simulink model "METI_CVT_Thermal_ver01_2015a"  (R2015a)
settings: Solver=ode8  SolverMode=SingleTasking  StartTime=0  StopTime=1204  FixedStep=sampling_time  RelTol=1e-3
PreLoadFcn:
  | init_setting;
values from neighbouring files (symbols this model uses):
  degC2K = 273.15    [METI_TRAMI_Thermal_ver01_Jmaab_PreLoad.m]    (also in init_setting_METI.m)
  K2degC = -273.15    [METI_TRAMI_Thermal_ver01_Jmaab_PreLoad.m]    (also in init_setting_METI.m)
  sampling_time = 0.0025    [METI_TRAMI_Thermal_ver01_Jmaab_PreLoad.m]
undefined symbols (not defined in the file or in its folder): ALT_CNT_ALT_OFF_RPM_HYS_rpm, ALT_CNT_ALT_ON_RPM_HYS_rpm, ALT_CNT_Alter_V_BASE_V, ALT_CNT_Alter_V_Kaisei_V, ALT_CNT_flag_disable_kaisei, ALT_CNT_V_Battely_Kudo_V, ALT_PNT_ALT_GDCurrent_A, ALT_PNT_ALT_GDVolt_V, ALT_PNT_Alter_limit_Current_V_table, ALT_PNT_Alter_limit_Current_V_table_x_rpm, ALT_PNT_Alter_trq_Nm_map, ALT_PNT_Alter_trq_Nm_map_x_rpm, ALT_PNT_Alter_trq_Nm_map_y_Current_A, ALT_PNT_Alter_trq_Nm_map_z_Volt_tgt_V, ALT_PNT_eta_pulley_alt, ALT_PNT_Gain_Alt_v_del, ALT_PNT_ratio_pulley_alt, ALT_PNT_Tau_Alternator_V_tgt_s, ALT_PNT_trq_alter_output_LL_Nm, BK_PNT_Pow_UL, BK_PNT_Tau_brake, Brk_LL, Brk_PGain, Brk_UL, BT_PNT_Lo_Capa_lo_batt_F, BT_PNT_Lo_ocv_SOC_lo_batt_OCV_V_table, BT_PNT_Lo_ocv_SOC_lo_batt_OCV_V_table_x_SOC, BT_PNT_Lo_R_lo_batt_ohm, BT_PNT_Lo_SOC_MAX_lo_batt, BT_PNT_Lo_SOC_MIN_lo_batt, BT_PNT_Lo_SOC_START_lo_batt, DF_PNT_DF_gear, DF_PNT_DFBlock2DFAir_Heat_Resi_KpW, DF_PNT_DFBlock_Heat_Capa_JpK, DF_PNT_DFBlock_Temp_ini_degC, DF_PNT_DFOil2DFBlock_Heat_Resi_KpW, DF_PNT_DFOil_Heat_Capa_JpK, DF_PNT_DFOil_Temp_ini_degC, DF_PNT_Driveshaft_damper, DF_PNT_Driveshaft_delta_radps_LL, DF_PNT_Driveshaft_delta_radps_UL, DF_PNT_Driveshaft_spring, DF_PNT_eta_DF, DF_PNT_Outtemp_degC, DF_PNT_TMBlock2DFBlock_Heat_Resi_KpW, Driver_Brake_Const1, Driver_Brake_Const3, Driver_Brake_Switch_Const2, Driver_Brk_sh, drivmode_ACC, drivmode_CONST, drivmode_GensokuKaisei, drivmode_GensokuRikko, drivmode_STOP, EL_PNT_R_bodyelec_lo_ohm, ENG_CNT_acc_idlestop, ENG_CNT_Accel_LL, ENG_CNT_Accel_UL, ENG_CNT_brak_idlestop, ENG_CNT_flag_idle_stop_exe ... (+133)
undefined symbols (not defined in the file): ACC_D_Gain, ACC_I_Gain, ACC_P_Gain
libraries: METI_Lib_vehicle_model x32, simulink x7, AZAPA_Lib_vehicle_model x1
(part 3 of 3)

== system METI_CVT_Thermal_ver01_2015a/Vehicle/TM_PNT/TC_PNT ==
  note: ロックアップクラッチ
  note: トルクコンバータ
  flag_Lockup : Inport
  omg_Slip_rpm : Inport  Port=2
  w_TM_PNT_in_radps : Inport  Port=3
  w_TM_PNT_in_radps2 : Inport  Port=4
  Gain : Gain  Gain=-1
  LU_Clutch : Subsystem
  P_cal : METI_Lib_vehicle_model/P_cal  Type_energy=回転運動  Type_output_energy=出力  Power_name=Po_  t_Workspace_Name=TM_PNT_TC_MECK_UP  P_VariableName=Po_TM_PNT_TC_MECK_UP  Across_VariableName=w_TM_PNT_TC_MECK_UP  Throgh_VariableName=tq_TM_PNT_TC_MECK_UP
  P_cal1 : METI_Lib_vehicle_model/P_cal  Type_energy=回転運動  Type_output_energy=出力  Power_name=Po_  t_Workspace_Name=TM_PNT_TC_MECK_DN  P_VariableName=Po_TM_PNT_TC_MECK_DN  Across_VariableName=w_TM_PNT_TC_MECK_DN  Throgh_VariableName=tq_TM_PNT_TC_MECK_DN
  P_cal2 : METI_Lib_vehicle_model/P_cal  Type_energy=回転運動  Type_output_energy=出力  Power_name=Po_  t_Workspace_Name=TM_PNT_LU_MECK_UP  P_VariableName=Po_TM_PNT_LU_MECK_UP  Across_VariableName=w_TM_PNT_LU_MECK_UP  Throgh_VariableName=tq_TM_PNT_LU_MECK_UP
  P_cal3 : METI_Lib_vehicle_model/P_cal  Type_energy=回転運動  Type_output_energy=出力  Power_name=Po_  t_Workspace_Name=TM_PNT_LU_MECK_DN  P_VariableName=Po_TM_PNT_LU_MECK_DN  Across_VariableName=w_TM_PNT_LU_MECK_DN  Throgh_VariableName=tq_TM_PNT_LU_MECK_DN
  Sum : Sum  Inputs=|++
  Sum1 : Sum  Inputs=|++
  T_C : Subsystem
  Terminator{,1..4} (5 alike) : Terminator
  trq_TM_PNT_in_Nm2 : Outport
  trq_TM_PNT_in_Nm1 : Outport  Port=2
  wires:
  T_C/2(trq_TC_Nm2) -> Sum/2, P_cal/2
  w_TM_PNT_in_radps/1 -> T_C/1(w_TM_PNT_in_radps1), P_cal/1, LU_Clutch/2(w_TM_PNT_in_radps1), P_cal2/1
  Sum/1 -> Gain/1
  T_C/1(trq_TC_Nm1) -> P_cal1/2, Sum1/2
  Sum1/1 -> trq_TM_PNT_in_Nm2/1
  w_TM_PNT_in_radps2/1 -> LU_Clutch/3(w_TM_PNT_in_radps2), P_cal1/1, P_cal3/1, T_C/2(w_TM_PNT_in_radps2)
  P_cal/1 -> Terminator/1
  P_cal1/1 -> Terminator1/1
  omg_Slip_rpm/1 -> Terminator3/1
  LU_Clutch/1(trq_LUC_Nm1) -> Sum/1, P_cal2/2
  LU_Clutch/2(trq_LUC_Nm2) -> Sum1/1, P_cal3/2
  flag_Lockup/1 -> LU_Clutch/1(LockUP_Signal)
  P_cal2/1 -> Terminator2/1
  P_cal3/1 -> Terminator4/1
  Gain/1 -> trq_TM_PNT_in_Nm1/1

== system METI_CVT_Thermal_ver01_2015a/Vehicle/TM_PNT/VR_PNT ==
  note: ギア比変換
  ratio_CVT : Inport
  trq_TM_PNT_in_Nm2 : Inport  Port=2
  w_TM_PNT_out_radps0 : Inport  Port=3
  T_TMTH_PNT_CVTF_dC : Inport  Port=4
  1-D Lookup Table : Lookup_n-D  NumberOfTableDimensions=1  BreakpointsForDimension1=TM_PNT_eta_CVT_x_CVTF_degC  Table=TM_PNT_eta_CVT  InternalRulePriority=Speed  RndMeth=Simplest  InputSameDT=on
  Goto1 : Goto  Commented=on  GotoTag=trq_Variator_Nm
  P_cal : METI_Lib_vehicle_model/P_cal  Type_energy=回転運動  Type_output_energy=損失  Power_name=Pl_  t_Workspace_Name=TM_PNT_Variator_MECK_LOSS  P_VariableName=Pl_TM_PNT_Variator_MECK_LOSS  Across_VariableName=w_TM_PNT_Variator_MECK_LOSS  Throgh_VariableName=tq_TM_PNT_Variator_MECK_LOSS
  Product : Product  RndMeth=Zero
  Product1 : Product  RndMeth=Zero
  Transfer Fcn : TransferFcn  Denominator=[TM_PNT_Tau_CVT_ratio_s 1]
  eta_cal_CVT : METI_Lib_vehicle_model/eta_cal_InHi
  trq_TM_PNT_out_Nm0 : Outport
  w_TM_PNT_in_radps2 : Outport  Port=2
  tag scope: tScope_CVTLoss=global
  wires:
  trq_TM_PNT_in_Nm2/1 -> eta_cal_CVT/2
  Product/1 -> w_TM_PNT_in_radps2/1, P_cal/1
  w_TM_PNT_out_radps0/1 -> Product/2
  ratio_CVT/1 -> Transfer Fcn/1
  Product1/1 -> Goto1/1, trq_TM_PNT_out_Nm0/1
  eta_cal_CVT/2 -> Product1/2
  P_cal/1 -> [tScope_CVTLoss]
  Transfer Fcn/1 -> Product1/1, Product/1
  1-D Lookup Table/1 -> eta_cal_CVT/1
  eta_cal_CVT/1 -> P_cal/2
  T_TMTH_PNT_CVTF_dC/1 -> 1-D Lookup Table/1

== system METI_CVT_Thermal_ver01_2015a/Driver/Caliculate_Opeining_Accel/FB/Filter ==
  In1 : Inport
  Gain3 : Gain  Gain=10
  Gain4 : Gain  Gain=0.1
  Rounding Function : Rounding  Operator=round
  Out1 : Outport
  wires:
  Rounding Function/1 -> Gain4/1
  In1/1 -> Gain3/1
  Gain3/1 -> Rounding Function/1
  Gain4/1 -> Out1/1

== system METI_CVT_Thermal_ver01_2015a/Driver/Caliculate_Opeining_Accel/FF/Air_Resistance ==
  V_tgt : Inport
  V_wind : Constant  Value=VL_PNT_V_wind
  cal_Air_resi1 : METI_Lib_vehicle_model/vehicle_model/cal_Air_resi  Vel_max=200
  F_air_resi : Outport
  wires:
  V_tgt/1 -> cal_Air_resi1/1
  V_wind/1 -> cal_Air_resi1/2
  cal_Air_resi1/1 -> F_air_resi/1

== system METI_CVT_Thermal_ver01_2015a/Driver/Caliculate_Opeining_Accel/FF/Cal_M_ENG_jiku2 ==
  note: 軸トルクマップ
  FF_trq_accel_Nm : Inport
  pre_n_eng_rpm : Inport  Port=2
  2-D Lookup Table : Lookup_n-D  BreakpointsForDimension1=ENG_trq_rev  BreakpointsForDimension2=ENG_rpm  Table=ENG_throttle_rev  ExtrapMethod=Clip  UseLastTableValue=on  RndMeth=Simplest  InputSameDT=on
  2-D Lookup Table1 : Lookup_n-D  BreakpointsForDimension1=ENG_PNT_trq_Nm_map_y_throttle  BreakpointsForDimension2=ENG_PNT_trq_Nm_map_x_rpm  Table=ENG_PNT_trq_Nm_map  ExtrapMethod=Clip  UseLastTableValue=on  RndMeth=Simplest  InputSameDT=on
  Constant : Constant  Value=0
  Subsystem : Subsystem
  Sum : Sum  Inputs=|++
  FF_open_accel_per : Outport
  wires:
  FF_trq_accel_Nm/1 -> Sum/1
  2-D Lookup Table/1 -> Subsystem/1(In1)
  pre_n_eng_rpm/1 -> 2-D Lookup Table/2, 2-D Lookup Table1/2
  Constant/1 -> 2-D Lookup Table1/1
  Sum/1 -> 2-D Lookup Table/1
  2-D Lookup Table1/1 -> Sum/2
  Subsystem/1(Out1) -> FF_open_accel_per/1

== system METI_CVT_Thermal_ver01_2015a/Driver/Caliculate_Opeining_Accel/FF/Inertial_Resistance ==
  V_tgt : Inport
  Constant : Constant  Value=M
  Derivative : Derivative
  Divide : Product  OutDataTypeStr=Inherit: Same as first input
  F_Inertia : Outport
  wires:
  Constant/1 -> Divide/2
  Derivative/1 -> Divide/1
  Divide/1 -> F_Inertia/1
  V_tgt/1 -> Derivative/1

== system METI_CVT_Thermal_ver01_2015a/Driver/Caliculate_Opeining_Accel/FF/Rolling_Resistance ==
  note: 20151211修正
      |
      | 空気抵抗と表現を統一する、ため
      | -1のGainを削除
  V_tgt : Inport
  cal_roll_resi1 : METI_Lib_vehicle_model/vehicle_model/cal_roll_resi  Myu_tire=myu  Vehicle_Mass=M  Gravi_acc=g
  F_rollresi : Outport
  wires:
  V_tgt/1 -> cal_roll_resi1/1
  cal_roll_resi1/1 -> F_rollresi/1

== system METI_CVT_Thermal_ver01_2015a/Vehicle/ALT_PNT/Subsystem/I_alt_cal ==
  target_volt_ALT_V : Inport
  volt_BT_PNT_Lo_V : Inport  Port=2
  rpm_alt : Inport  Port=3
  Add : Sum
  Cal_I_alt_P_control : Subsystem
  Cal_I_alt_base : Subsystem
  Constant : Constant  Value=12
  Constant4 : Constant  Value=0
  Limit_Current_Max : Lookup_n-D  NumberOfTableDimensions=1  BreakpointsForDimension1=ALT_PNT_Alter_limit_Current_V_table_x_rpm  Table=ALT_PNT_Alter_limit_Current_V_table  ExtrapMethod=Clip  UseLastTableValue=on  RndMeth=Simplest  InputSameDT=on
  MinMax2 : MinMax  Function=max  Inputs=2
  Sum1 : Sum  Inputs=|+-
  Sum2 : Sum  Inputs=-+|
  電圧比較 : MinMax  Inputs=2
  I_alt : Outport
  wires:
  target_volt_ALT_V/1 -> Sum1/1, Sum2/2
  volt_BT_PNT_Lo_V/1 -> Sum2/1
  rpm_alt/1 -> Limit_Current_Max/1
  Constant4/1 -> MinMax2/2
  Limit_Current_Max/1 -> MinMax2/1  "I_limit_ALT"
  電圧比較/1 -> I_alt/1
  Add/1 -> 電圧比較/2
  Sum2/1 -> Cal_I_alt_P_control/1(V_delt_tgt)
  MinMax2/1 -> 電圧比較/1
  Constant/1 -> Sum1/2
  Sum1/1 -> Cal_I_alt_base/1(V_delt_tgt)
  Cal_I_alt_P_control/1(I_alt_base) -> Add/1
  Cal_I_alt_base/1(I_alt_base) -> Add/2

== system METI_CVT_Thermal_ver01_2015a/Vehicle/ALT_PNT/Subsystem/Torque_Guard ==
  current_ALT_PNT_A : Inport
  V_ALT_PNT : Inport  Port=2
  n_ROT_slavepulley12_rpm : Inport  Port=3
  ALT_GDCurrent : Inport  Port=4
  ALT_GDVolt : Inport  Port=5
  Caliculate_Axes_Torque1 : Lookup_n-D  NumberOfTableDimensions=3  BreakpointsForDimension1=ALT_PNT_Alter_trq_Nm_map_x_rpm  BreakpointsForDimension2=ALT_PNT_Alter_trq_Nm_map_y_Current_A  BreakpointsForDimension3=ALT_PNT_Alter_trq_Nm_map_z_Volt_tgt_V  Table=ALT_PNT_Alter_trq_Nm_map  RndMeth=Simplest  InputSameDT=on
  Caliculate_Axes_Torque2 : Lookup_n-D  NumberOfTableDimensions=3  BreakpointsForDimension1=ALT_PNT_Alter_trq_Nm_map_x_rpm  BreakpointsForDimension2=ALT_PNT_Alter_trq_Nm_map_y_Current_A  BreakpointsForDimension3=ALT_PNT_Alter_trq_Nm_map_z_Volt_tgt_V  Table=ALT_PNT_Alter_trq_Nm_map  RndMeth=Simplest  InputSameDT=on
  Constant3 : Constant  Value=ALT_PNT_trq_alter_output_LL_Nm
  MinMax : MinMax  Inputs=2
  MinMax1 : MinMax  Function=max  Inputs=2
  trq_trqsource : Outport
  wires:
  ALT_GDCurrent/1 -> Caliculate_Axes_Torque2/2
  Caliculate_Axes_Torque2/1 -> MinMax/2
  MinMax/1 -> MinMax1/1
  Caliculate_Axes_Torque1/1 -> MinMax/1
  Constant3/1 -> MinMax1/2
  ALT_GDVolt/1 -> Caliculate_Axes_Torque2/3
  MinMax1/1 -> trq_trqsource/1
  V_ALT_PNT/1 -> Caliculate_Axes_Torque1/3
  current_ALT_PNT_A/1 -> Caliculate_Axes_Torque1/2
  n_ROT_slavepulley12_rpm/1 -> Caliculate_Axes_Torque2/1, Caliculate_Axes_Torque1/1

== system METI_CVT_Thermal_ver01_2015a/Vehicle/BT_LO_PNT/Cal_SOC/Subsystem4 ==
  In1 : Inport
  In2 : Inport  Port=2
  To Workspace : ToWorkspace  VariableName=SOC_LoBat  SampleTime=-1
      settings: Decimation=num_tws_mabiki
  To Workspace1 : ToWorkspace  VariableName=Asec_LoBat  SampleTime=-1
      settings: Decimation=num_tws_mabiki
  wires:
  In1/1 -> To Workspace/1
  In2/1 -> To Workspace1/1

== system METI_CVT_Thermal_ver01_2015a/Vehicle/ENG_CNT/Caliculate_Idle_Speed/Subsystem ==
  del_omg_engine : Inport
  flag_idle_fb : Inport  Port=2
  Gain : Gain  Gain=ENG_CNT_gain_p_per_isc
  Logical Operator1 : Logic  Operator=NOT  AllPortsSameDT=off  OutDataTypeStr=boolean
  Memory : Memory  X0=4
  Saturation : Saturate  UpperLimit=ENG_CNT_per_isc_max  LowerLimit=ENG_CNT_per_isc_min
  Switch : Switch  Criteria=u2 > Threshold  Threshold=0.5
  per_isc_[%] : Outport
  wires:
  Switch/1 -> Saturation/1
  flag_idle_fb/1 -> Logical Operator1/1
  Gain/1 -> Switch/3
  Memory/1 -> Switch/1
  Saturation/1 -> per_isc_[%]/1, Memory/1
  del_omg_engine/1 -> Gain/1
  Logical Operator1/1 -> Switch/2

== system METI_CVT_Thermal_ver01_2015a/Vehicle/ENG_CNT/Caliculate_Idle_Speed/Subsystem1 ==
  note: アイドル回転数時のFB
  omg_tgt_idle : Inport
  n_eng_rpm : Inport  Port=2
  per_throttle_base : Inport  Port=3
  flag_Lockup : Inport  Port=4
  flag_IdleStop : Inport  Port=5
  Logical Operator : Logic  Operator=OR  AllPortsSameDT=off  OutDataTypeStr=boolean
  Logical Operator1 : Logic  Operator=NOT  AllPortsSameDT=off  OutDataTypeStr=boolean
  Logical Operator2 : Logic  Inputs=3  AllPortsSameDT=off  OutDataTypeStr=boolean
  Logical Operator3 : Logic  Operator=NOT  AllPortsSameDT=off  OutDataTypeStr=boolean
  Logical Operator4 : Logic  Operator=NOT  AllPortsSameDT=off  OutDataTypeStr=boolean
  Logical Operator5 : Logic  AllPortsSameDT=off  OutDataTypeStr=boolean
  Relational Operator : RelationalOperator  Operator=<  OutDataTypeStr=boolean
  Relational Operator2 : RelationalOperator  Operator=>  OutDataTypeStr=boolean
  per_throttle_isc_fb : Constant  Value=ENG_CNT_per_throttle_isc_fb
  flag_idle_fb : Outport
  wires:
  per_throttle_base/1 -> Relational Operator/1
  per_throttle_isc_fb/1 -> Relational Operator/2
  Relational Operator2/1 -> Logical Operator2/1
  Relational Operator/1 -> Logical Operator1/1, Logical Operator5/1
  Logical Operator1/1 -> Logical Operator2/2
  Logical Operator5/1 -> Logical Operator/2
  flag_Lockup/1 -> Logical Operator3/1
  Logical Operator3/1 -> Logical Operator2/3
  Logical Operator2/1 -> Logical Operator/1
  omg_tgt_idle/1 -> Relational Operator2/1
  n_eng_rpm/1 -> Relational Operator2/2
  flag_IdleStop/1 -> Logical Operator4/1
  Logical Operator4/1 -> Logical Operator5/2
  Logical Operator/1 -> flag_idle_fb/1

== system METI_CVT_Thermal_ver01_2015a/Vehicle/ENG_PNT/Cal_FuelComsunption/Not_cal1 ==
  In1 : Inport
  Constant : Constant  Value=0
  Constant1 : Constant
  Switch : Switch  Criteria=u2 > Threshold  Threshold=0.5
  Out1 : Outport
  wires:
  Constant1/1 -> Switch/3
  Constant/1 -> Switch/1
  Switch/1 -> Out1/1
  In1/1 -> Switch/2

== system METI_CVT_Thermal_ver01_2015a/Vehicle/ENG_PNT/Cal_FuelComsunption/Not_cal2 ==
  In1 : Inport
  Constant : Constant  Value=0
  Constant1 : Constant
  Switch : Switch  Criteria=u2 > Threshold  Threshold=0.5
  Out1 : Outport
  wires:
  In1/1 -> Switch/2
  Switch/1 -> Out1/1
  Constant/1 -> Switch/1
  Constant1/1 -> Switch/3

== system METI_CVT_Thermal_ver01_2015a/Vehicle/ENG_PNT/Cal_trq_ENG_jiku/Not_cal ==
  In1 : Inport
  Constant : Constant  Value=0
  Constant1 : Constant
  Switch : Switch  Criteria=u2 > Threshold  Threshold=0.5
  Out1 : Outport
  wires:
  In1/1 -> Switch/2
  Switch/1 -> Out1/1
  Constant/1 -> Switch/1
  Constant1/1 -> Switch/3

== system METI_CVT_Thermal_ver01_2015a/Vehicle/ENG_PNT/Cal_trq_ENG_jiku/Not_cal1 ==
  In1 : Inport
  Constant : Constant  Value=0
  Constant1 : Constant
  Switch : Switch  Criteria=u2 > Threshold  Threshold=0.5
  Out1 : Outport
  wires:
  Constant1/1 -> Switch/3
  Constant/1 -> Switch/1
  Switch/1 -> Out1/1
  In1/1 -> Switch/2

== system METI_CVT_Thermal_ver01_2015a/Vehicle/PTTH_PNT/DFTH_PNT/DFBlock_Heat_Capacity ==
  PHI_DFBlock3_W : Inport
  PHI_DFBlock2_W : Inport  Port=2
  PHI_DFBlock1_W : Inport  Port=3
  Add : Sum  Inputs=+++
  Add1 : Sum
  Constant : Constant  Value=DF_PNT_DFBlock_Heat_Capa_JpK
  Constant1 : Constant  Value=DF_PNT_DFBlock_Temp_ini_degC
  Divide : Product  Inputs=/*
  Integrator : Integrator
  degC->K : Subsystem
  T_DFBlock2_K : Outport
  T_DFBlock3_K : Outport  Port=2
  T_DFBlock1_K : Outport  Port=3
  wires:
  PHI_DFBlock1_W/1 -> Add/1
  Constant/1 -> Divide/1
  Add/1 -> Divide/2
  Divide/1 -> Integrator/1
  Integrator/1 -> Add1/2
  Add1/1 -> T_DFBlock1_K/1, T_DFBlock3_K/1, T_DFBlock2_K/1
  PHI_DFBlock2_W/1 -> Add/2
  PHI_DFBlock3_W/1 -> Add/3
  Constant1/1 -> degC->K/1(degC)
  degC->K/1(K) -> Add1/1

== system METI_CVT_Thermal_ver01_2015a/Vehicle/PTTH_PNT/DFTH_PNT/DFOil2DFBlock_Heat_Resistance ==
  T_DFOil_Resi2_K : Inport
  T_DFBlock_Resi_K : Inport  Port=2
  Add : Sum  Inputs=+-
  Constant : Constant  Value=DF_PNT_DFOil2DFBlock_Heat_Resi_KpW
  Divide : Product  Inputs=*/
  Gain : Gain  Gain=-1
  Gain1 : Gain
  PHI_DFOil_Resi2_W : Outport
  PHI_DFBlock_Resi_W : Outport  Port=2
  wires:
  Constant/1 -> Divide/2
  Add/1 -> Divide/1
  Divide/1 -> Gain/1, Gain1/1
  Gain/1 -> PHI_DFOil_Resi2_W/1
  T_DFOil_Resi2_K/1 -> Add/1
  T_DFBlock_Resi_K/1 -> Add/2
  Gain1/1 -> PHI_DFBlock_Resi_W/1

== system METI_CVT_Thermal_ver01_2015a/Vehicle/PTTH_PNT/DFTH_PNT/DFOil_Heat_Capacity ==
  PHI_DFOil2_W : Inport
  PHI_DFOil1_W : Inport  Port=2
  Add : Sum
  Add1 : Sum
  Constant : Constant  Value=DF_PNT_DFOil_Heat_Capa_JpK
  Constant1 : Constant  Value=DF_PNT_DFOil_Temp_ini_degC
  Divide : Product  Inputs=/*
  Integrator : Integrator
  degC->K : Subsystem
  T_DFOil2_K : Outport
  T_DFOil1_K : Outport  Port=2
  wires:
  PHI_DFOil2_W/1 -> Add/2
  PHI_DFOil1_W/1 -> Add/1
  Constant/1 -> Divide/1
  Add/1 -> Divide/2
  Divide/1 -> Integrator/1
  Integrator/1 -> Add1/2
  Add1/1 -> T_DFOil1_K/1, T_DFOil2_K/1
  Constant1/1 -> degC->K/1(degC)
  degC->K/1(K) -> Add1/1

== system METI_CVT_Thermal_ver01_2015a/Vehicle/PTTH_PNT/DFTH_PNT/ENGBlock2Air_Heat_Resistance ==
  T_DFBlock_Resi_K : Inport
  T_DF_Air_Resi_K : Inport  Port=2
  Add : Sum  Inputs=+-
  Constant : Constant  Value=DF_PNT_DFBlock2DFAir_Heat_Resi_KpW
  Divide : Product  Inputs=*/
  Gain : Gain  Gain=-1
  Gain1 : Gain
  PHI_DFBlock_Resi_W : Outport
  PHI_DF_Air_Resi_W : Outport  Port=2
  wires:
  Constant/1 -> Divide/2
  Add/1 -> Divide/1
  Divide/1 -> Gain/1, Gain1/1
  Gain/1 -> PHI_DFBlock_Resi_W/1
  T_DFBlock_Resi_K/1 -> Add/1
  T_DF_Air_Resi_K/1 -> Add/2
  Gain1/1 -> PHI_DF_Air_Resi_W/1

== system METI_CVT_Thermal_ver01_2015a/Vehicle/PTTH_PNT/DFTH_PNT/TMBlock2DFBlock_Heat_Resistance ==
  T_DFBlock_Resi_K : Inport
  T_TMBlock_Resi_K : Inport  Port=2
  Add : Sum  Inputs=+-
  Constant : Constant  Value=DF_PNT_TMBlock2DFBlock_Heat_Resi_KpW
  Divide : Product  Inputs=*/
  Gain : Gain  Gain=-1
  Gain1 : Gain
  PHI_DFBlock_Resi_W : Outport
  PHI_TMBlock_Resi_W : Outport  Port=2
  wires:
  Constant/1 -> Divide/2
  Add/1 -> Divide/1
  Divide/1 -> Gain/1, Gain1/1
  Gain/1 -> PHI_TMBlock_Resi_W/1
  T_TMBlock_Resi_K/1 -> Add/1
  T_DFBlock_Resi_K/1 -> Add/2
  Gain1/1 -> PHI_DFBlock_Resi_W/1

== system METI_CVT_Thermal_ver01_2015a/Vehicle/PTTH_PNT/ENGTH_PNT/Coolant_Heat_Capacity ==
  PHI_Coolant4_W : Inport
  PHI_Coolant1_W : Inport  Port=2
  PHI_Coolant3_W : Inport  Port=3
  PHI_Coolant2_W : Inport  Port=4
  Add : Sum  Inputs=++++
  Add1 : Sum
  Constant : Constant  Value=ENG_PNT_Coolant_Heat_Capa_JpK
  Constant1 : Constant  Value=ENG_PNT_Coolant_Temp_ini_degC
  Divide : Product  Inputs=/*
  Integrator : Integrator
  degC->K : Subsystem
  T_Coolant1_K : Outport
  T_Coolant4_K : Outport  Port=2
  T_Coolant2_K : Outport  Port=3
  T_Coolant3_K : Outport  Port=4
  wires:
  PHI_Coolant2_W/1 -> Add/4
  PHI_Coolant1_W/1 -> Add/1
  Constant/1 -> Divide/1
  Add/1 -> Divide/2
  Divide/1 -> Integrator/1
  Integrator/1 -> Add1/2
  Add1/1 -> T_Coolant3_K/1, T_Coolant2_K/1, T_Coolant4_K/1, T_Coolant1_K/1
  PHI_Coolant3_W/1 -> Add/2
  PHI_Coolant4_W/1 -> Add/3
  degC->K/1(K) -> Add1/1
  Constant1/1 -> degC->K/1(degC)

== system METI_CVT_Thermal_ver01_2015a/Vehicle/PTTH_PNT/ENGTH_PNT/Cylinder_Head2Coolant_Heat_Resistance ==
  T_Coolant_Resi1_K : Inport
  Qv_Coolant_m3ps : Inport  Port=2
  T_Cylinder_Head_Resi2_K : Inport  Port=3
  1-D Lookup Table : Lookup_n-D  NumberOfTableDimensions=1  BreakpointsForDimension1=ENG_PNT_Cylinder_Head2Coolant_Heat_Resi_x_qv_Coolant  Table=ENG_PNT_Cylinder_Head2Coolant_Heat_Resi_KpW  InternalRulePriority=Speed  RndMeth=Simplest  InputSameDT=on
  Add : Sum  Inputs=+-
  Divide : Product  Inputs=*/
  Gain : Gain  Gain=-1
  Gain1 : Gain
  PHI_Coolant_Resi1_W : Outport
  PHI_Cylinder_Head_Resi2_W : Outport  Port=2
  wires:
  T_Cylinder_Head_Resi2_K/1 -> Add/1
  T_Coolant_Resi1_K/1 -> Add/2
  1-D Lookup Table/1 -> Divide/2
  Add/1 -> Divide/1
  Divide/1 -> Gain/1, Gain1/1
  Gain/1 -> PHI_Cylinder_Head_Resi2_W/1
  Gain1/1 -> PHI_Coolant_Resi1_W/1
  Qv_Coolant_m3ps/1 -> 1-D Lookup Table/1

== system METI_CVT_Thermal_ver01_2015a/Vehicle/PTTH_PNT/ENGTH_PNT/ENGBlock2Air_Heat_Resistance ==
  T_ENGBlock_Resi3_K : Inport
  T_ENG_Air_Resi1_K : Inport  Port=2
  Add : Sum  Inputs=+-
  Constant : Constant  Value=ENG_PNT_ENGBlock2ENGAir_Heat_Resi_KpW
  Divide : Product  Inputs=*/
  Gain : Gain  Gain=-1
  Gain1 : Gain
  PHI_ENGBlock_Resi3_W : Outport
  PHI_ENG_Air_Resi1_W : Outport  Port=2
  wires:
  Constant/1 -> Divide/2
  Add/1 -> Divide/1
  Divide/1 -> Gain1/1, Gain/1
  Gain/1 -> PHI_ENGBlock_Resi3_W/1
  T_ENGBlock_Resi3_K/1 -> Add/1
  T_ENG_Air_Resi1_K/1 -> Add/2
  Gain1/1 -> PHI_ENG_Air_Resi1_W/1

== system METI_CVT_Thermal_ver01_2015a/Vehicle/PTTH_PNT/ENGTH_PNT/ENGBlock2Coolant_Heat_Resistance ==
  T_Coolant_Resi4_K : Inport
  T_ENGBlock_Resi1_K : Inport  Port=2
  Add : Sum  Inputs=+-
  Constant : Constant  Value=ENG_PNT_Coolant2ENGBlock_Heat_Resi_KpW
  Divide : Product  Inputs=*/
  Gain : Gain  Gain=-1
  Gain1 : Gain
  PHI_Coolant_Resi4_W : Outport
  PHI_ENGBlock_Resi1_W : Outport  Port=2
  wires:
  Constant/1 -> Divide/2
  Add/1 -> Divide/1
  Divide/1 -> Gain1/1, Gain/1
  Gain/1 -> PHI_Coolant_Resi4_W/1
  T_Coolant_Resi4_K/1 -> Add/1
  T_ENGBlock_Resi1_K/1 -> Add/2
  Gain1/1 -> PHI_ENGBlock_Resi1_W/1

== system METI_CVT_Thermal_ver01_2015a/Vehicle/PTTH_PNT/ENGTH_PNT/ENGBlock_Heat_Capacity ==
  PHI_ENGBlock3_W : Inport
  PHI_ENGBlock1_W : Inport  Port=2
  PHI_ENGBlock2_W : Inport  Port=3
  Add : Sum  Inputs=+++
  Add1 : Sum
  Constant : Constant  Value=ENG_PNT_ENGBlock_Heat_Capa_JpK
  Constant1 : Constant  Value=ENG_PNT_ENGBlock_Temp_ini_degC
  Divide : Product  Inputs=/*
  Integrator : Integrator
  degC->K : Subsystem
  T_ENGBlock3_K : Outport
  T_ENGBlock2_K : Outport  Port=2
  T_ENGBlock1_K : Outport  Port=3
  wires:
  PHI_ENGBlock2_W/1 -> Add/3
  PHI_ENGBlock1_W/1 -> Add/1
  Constant/1 -> Divide/1
  Add/1 -> Divide/2
  Divide/1 -> Integrator/1
  Integrator/1 -> Add1/2
  Add1/1 -> T_ENGBlock2_K/1, T_ENGBlock1_K/1, T_ENGBlock3_K/1
  PHI_ENGBlock3_W/1 -> Add/2
  Constant1/1 -> degC->K/1(degC)
  degC->K/1(K) -> Add1/1

== system METI_CVT_Thermal_ver01_2015a/Vehicle/PTTH_PNT/ENGTH_PNT/ENGOil2Coolant_Heat_Resistance ==
  T_ENGOil_Resi2_K : Inport
  T_Coolant_Resi3_K : Inport  Port=2
  Add : Sum  Inputs=+-
  Constant : Constant  Value=ENG_PNT_ENGOil2Coolant_Heat_Resi_KpW
  Divide : Product  Inputs=*/
  Gain : Gain  Gain=-1
  Gain1 : Gain
  PHI_ENGOil_Resi2_W : Outport
  PHI_Coolant_Resi3_W : Outport  Port=2
  wires:
  T_ENGOil_Resi2_K/1 -> Add/1
  T_Coolant_Resi3_K/1 -> Add/2
  Constant/1 -> Divide/2
  Add/1 -> Divide/1
  Divide/1 -> Gain/1, Gain1/1
  Gain/1 -> PHI_ENGOil_Resi2_W/1
  Gain1/1 -> PHI_Coolant_Resi3_W/1

== system METI_CVT_Thermal_ver01_2015a/Vehicle/PTTH_PNT/ENGTH_PNT/ENGOil_Heat_Capacity ==
  PHI_ENGOil2_W : Inport
  PHI_ENGOil1_W : Inport  Port=2
  Add : Sum
  Add1 : Sum
  Constant : Constant  Value=ENG_PNT_ENGOil_Heat_Capa_JpK
  Constant1 : Constant  Value=ENG_PNT_ENGOil_Temp_ini_degC
  Divide : Product  Inputs=/*
  Integrator : Integrator
  degC->K : Subsystem
  T_ENGOil2_K : Outport
  T_ENGOil1_K : Outport  Port=2
  wires:
  PHI_ENGOil2_W/1 -> Add/2
  PHI_ENGOil1_W/1 -> Add/1
  Constant/1 -> Divide/1
  Add/1 -> Divide/2
  Divide/1 -> Integrator/1
  Integrator/1 -> Add1/2
  Add1/1 -> T_ENGOil2_K/1, T_ENGOil1_K/1
  Constant1/1 -> degC->K/1(degC)
  degC->K/1(K) -> Add1/1

== system METI_CVT_Thermal_ver01_2015a/Vehicle/PTTH_PNT/ENGTH_PNT/ENGOil_Heat_Capacity1 ==
  PHI_Cylinder_Head1_W : Inport
  PHI_Cylinder_Head2_W : Inport  Port=2
  Add : Sum
  Add1 : Sum
  Constant : Constant  Value=ENG_PNT_Cylinder_Head_Heat_Capa_JpK
  Constant1 : Constant  Value=ENG_PNT_Cylinder_Head_Temp_ini_degC
  Divide : Product  Inputs=/*
  Integrator : Integrator
  degC->K : Subsystem
  T_Cylinder_Head1_K : Outport
  T_Cylinder_Head2_K : Outport  Port=2
  wires:
  PHI_Cylinder_Head2_W/1 -> Add/2
  PHI_Cylinder_Head1_W/1 -> Add/1
  Constant/1 -> Divide/1
  Add/1 -> Divide/2
  Divide/1 -> Integrator/1
  Integrator/1 -> Add1/2
  Add1/1 -> T_Cylinder_Head2_K/1, T_Cylinder_Head1_K/1
  Constant1/1 -> degC->K/1(degC)
  degC->K/1(K) -> Add1/1

== system METI_CVT_Thermal_ver01_2015a/Vehicle/PTTH_PNT/ENGTH_PNT/Water_Pump ==
  ENG_PNT_Voltage_WP_V : Inport
  1-D Lookup Table : Lookup_n-D  NumberOfTableDimensions=1  BreakpointsForDimension1=ENG_PNT_Qv_Water_Pump_x_V_WP  Table=ENG_PNT_Qv_Water_Pump_m3ps  InternalRulePriority=Speed  RndMeth=Simplest  InputSameDT=on
  Qv_Coolant_m3ps : Outport
  wires:
  ENG_PNT_Voltage_WP_V/1 -> 1-D Lookup Table/1
  1-D Lookup Table/1 -> Qv_Coolant_m3ps/1

== system METI_CVT_Thermal_ver01_2015a/Vehicle/PTTH_PNT/RDTH_PNT/ENGBlock2Coolant_Heat_Resistance ==
  T_RDCoolant_Resi1_K : Inport
  T_Thermostat_Resi1_K : Inport  Port=2
  1-D Lookup Table : Lookup_n-D  NumberOfTableDimensions=1  BreakpointsForDimension1=RD_PNT_Thermostat_Heat_Resi_KpW_T_Coolant  Table=RD_PNT_Thermostat_Heat_Resi_KpW  InternalRulePriority=Speed  RndMeth=Simplest  InputSameDT=on
  Add : Sum  Inputs=+-
  Divide : Product  Inputs=*/
  Gain : Gain  Gain=-1
  Gain1 : Gain
  K->degC : Subsystem
  PHI_RDCoolant_Resi1_W : Outport
  PHI_Thermostat_Resi1_W : Outport  Port=2
  tag scope: RD_PNT_Thermostat_Heat_Resi_KpW=global
  wires:
  Add/1 -> Divide/1
  Divide/1 -> Gain/1, Gain1/1
  Gain/1 -> PHI_Thermostat_Resi1_W/1
  T_Thermostat_Resi1_K/1 -> Add/1, K->degC/1(K)
  T_RDCoolant_Resi1_K/1 -> Add/2
  Gain1/1 -> PHI_RDCoolant_Resi1_W/1
  K->degC/1(degC) -> 1-D Lookup Table/1
  1-D Lookup Table/1 -> [RD_PNT_Thermostat_Heat_Resi_KpW], Divide/2

== system METI_CVT_Thermal_ver01_2015a/Vehicle/PTTH_PNT/RDTH_PNT/RDCoolant2Air_Heat_Resistance ==
  T_RD_Air_Resi_K : Inport
  "RD_PNT_RDCore_Heat_Resi_KpW " : Inport  Port=2
  T_RDCoolant_Resi2_K : Inport  Port=3
  Add : Sum  Inputs=+-
  Divide : Product  Inputs=*/
  Gain : Gain  Gain=-1
  Gain1 : Gain
  PHI_RD_Air_Resi1_W : Outport
  PHI_RDCoolant_Resi2_W : Outport  Port=2
  wires:
  "RD_PNT_RDCore_Heat_Resi_KpW "/1 -> Divide/2
  Add/1 -> Divide/1
  Divide/1 -> Gain/1, Gain1/1
  Gain/1 -> PHI_RDCoolant_Resi2_W/1
  T_RDCoolant_Resi2_K/1 -> Add/1
  T_RD_Air_Resi_K/1 -> Add/2
  Gain1/1 -> PHI_RD_Air_Resi1_W/1

== system METI_CVT_Thermal_ver01_2015a/Vehicle/PTTH_PNT/RDTH_PNT/RDCoolant_Heat_Capacity ==
  PHI_RDCoolant1_W : Inport
  PHI_RDCoolant2_W : Inport  Port=2
  Add : Sum
  Add1 : Sum
  Constant : Constant  Value=RD_PNT_RDCoolant_Heat_Capa_JpK
  Constant1 : Constant  Value=RD_PNT_RDCoolant_Temp_ini_degC
  Divide : Product  Inputs=/*
  Integrator : Integrator
  degC->K : Subsystem
  T_RDCoolant1_K : Outport
  T_RDCoolant2_K : Outport  Port=2
  wires:
  PHI_RDCoolant2_W/1 -> Add/2
  PHI_RDCoolant1_W/1 -> Add/1
  Constant/1 -> Divide/1
  Add/1 -> Divide/2
  Divide/1 -> Integrator/1
  Integrator/1 -> Add1/2
  Add1/1 -> T_RDCoolant2_K/1, T_RDCoolant1_K/1
  Constant1/1 -> degC->K/1(degC)
  degC->K/1(K) -> Add1/1

== system METI_CVT_Thermal_ver01_2015a/Vehicle/PTTH_PNT/RDTH_PNT/RD_Core_Heat_Resi_Calc ==
  note: ラジエターファンの動作で
      | 発生する風速
  note: 車両の走行によって
      | ラジエターグリルに発生する風速
  note: ラジエターファンの動作で
      | ラジエターコアに当たる風量
  note: 車両の走行によって
      | ラジエターコアに当たる風量
  RD_PNT_Voltage_RDFan_V : Inport
  v_VL_PNT_kmph : Inport  Port=2
  1-D Lookup Table : Lookup_n-D  NumberOfTableDimensions=1  BreakpointsForDimension1=RD_PNT_RDCore_Heat_Resi_KpW_x_Wind_m3ps  Table=RD_PNT_RDCore_Heat_Resi_KpW  InternalRulePriority=Speed  RndMeth=Simplest  InputSameDT=on
  1-D Lookup Table1 : Lookup_n-D  NumberOfTableDimensions=1  BreakpointsForDimension1=RD_PNT_v_RDFan_Wind_vel_mps_x_V_RDFan  Table=RD_PNT_v_RDFan_Wind_vel_mps  InternalRulePriority=Speed  RndMeth=Simplest  InputSameDT=on
  Abs : Abs
  Add : Sum
  Constant : Constant  Value=RD_PNT_RDFan_area_m2
  Constant1 : Constant  Value=RD_PNT_RDGrill_area_m2
  Product : Product
  Product1 : Product
  gain1 : Gain  Gain=kmph2mps
  "RD_PNT_RDCore_Heat_Resi_KpW " : Outport
  wires:
  RD_PNT_Voltage_RDFan_V/1 -> 1-D Lookup Table1/1
  Constant/1 -> Product/2
  v_VL_PNT_kmph/1 -> gain1/1
  Constant1/1 -> Product1/2
  Product/1 -> Add/1
  Product1/1 -> Add/2
  Add/1 -> Abs/1
  1-D Lookup Table/1 -> "RD_PNT_RDCore_Heat_Resi_KpW "/1
  Abs/1 -> 1-D Lookup Table/1
  1-D Lookup Table1/1 -> Product/1
  gain1/1 -> Product1/1

== system METI_CVT_Thermal_ver01_2015a/Vehicle/PTTH_PNT/TMTH_PNT/CVTF2Coolant_Heat_Resistance ==
  note: エネルギーの
      | 向きの定義（仮）
      | ← ←←
  T_CVTF_Resi2_K : Inport
  R_CVTF_warmer_tgt_KpW : Inport  Port=2
  T_Coolant_Resi2_K : Inport  Port=3
  Add : Sum  Inputs=+-
  Divide : Product  Inputs=*/
  Gain : Gain  Gain=-1
  Gain1 : Gain  Gain=-1
  PHI_Coolant_Resi2_W : Outport
  PHI_CVTF_Resi2_W : Outport  Port=2
  wires:
  R_CVTF_warmer_tgt_KpW/1 -> Divide/2
  Add/1 -> Divide/1
  Divide/1 -> Gain/1, Gain1/1
  T_Coolant_Resi2_K/1 -> Add/2
  T_CVTF_Resi2_K/1 -> Add/1
  Gain/1 -> PHI_CVTF_Resi2_W/1
  Gain1/1 -> PHI_Coolant_Resi2_W/1

== system METI_CVT_Thermal_ver01_2015a/Vehicle/PTTH_PNT/TMTH_PNT/CVTF2TMBlock_Heat_Resistance ==
  T_CVTF_Resi4_K : Inport
  T_TMBlock_Resi1_K : Inport  Port=2
  Add : Sum  Inputs=+-
  Constant : Constant  Value=TM_PNT_CVTF2TMBlock_Heat_Resi_KpW
  Divide : Product  Inputs=*/
  Gain : Gain  Gain=-1
  Gain1 : Gain
  PHI_CVTF_Resi4_W : Outport
  PHI_TMBlock_Resi1_W : Outport  Port=2
  wires:
  Constant/1 -> Divide/2
  Add/1 -> Divide/1
  Divide/1 -> Gain/1, Gain1/1
  Gain/1 -> PHI_CVTF_Resi4_W/1
  T_CVTF_Resi4_K/1 -> Add/1
  T_TMBlock_Resi1_K/1 -> Add/2
  Gain1/1 -> PHI_TMBlock_Resi1_W/1

== system METI_CVT_Thermal_ver01_2015a/Vehicle/PTTH_PNT/TMTH_PNT/CVTF_Heat_Capacity ==
  PHI_CVTF4_W : Inport
  PHI_CVTF1_W : Inport  Port=2
  PHI_CVT2_W : Inport  Port=3
  Add : Sum  Inputs=+++
  Add1 : Sum
  Constant : Constant  Value=TM_PNT_CVTF_Heat_Capa_JpK
  Constant1 : Constant  Value=TM_PNT_CVTF_Temp_ini_degC
  Divide : Product  Inputs=/*
  Integrator : Integrator
  degC->K : Subsystem
  T_CVTF4_K : Outport
  T_CVTF2_K : Outport  Port=2
  T_CVTF1_K : Outport  Port=3
  wires:
  PHI_CVT2_W/1 -> Add/3
  PHI_CVTF1_W/1 -> Add/1
  Constant/1 -> Divide/1
  Add/1 -> Divide/2
  Divide/1 -> Integrator/1
  Integrator/1 -> Add1/2
  Add1/1 -> T_CVTF1_K/1, T_CVTF2_K/1, T_CVTF4_K/1
  PHI_CVTF4_W/1 -> Add/2
  Constant1/1 -> degC->K/1(degC)
  degC->K/1(K) -> Add1/1

== system METI_CVT_Thermal_ver01_2015a/Vehicle/PTTH_PNT/TMTH_PNT/ENGBlock2TMBlock_Heat_Resistance ==
  T_TMBlock_Resi2_K : Inport
  T_ENGBlock_Resi2_K : Inport  Port=2
  Add : Sum  Inputs=+-
  Constant : Constant  Value=TM_PNT_ENGBlock2TMBlock_Heat_Resi_KpW
  Divide : Product  Inputs=*/
  Gain : Gain  Gain=-1
  Gain1 : Gain
  PHI_TMBlock_Resi2_W : Outport
  PHI_ENGBlock_Resi2_W : Outport  Port=2
  wires:
  Constant/1 -> Divide/2
  Add/1 -> Divide/1
  Divide/1 -> Gain1/1, Gain/1
  Gain/1 -> PHI_ENGBlock_Resi2_W/1
  T_ENGBlock_Resi2_K/1 -> Add/1
  T_TMBlock_Resi2_K/1 -> Add/2
  Gain1/1 -> PHI_TMBlock_Resi2_W/1

== system METI_CVT_Thermal_ver01_2015a/Vehicle/PTTH_PNT/TMTH_PNT/TMBlock2Air_Heat_Resistance ==
  T_TMBlock_Resi3_K : Inport
  T_TM_Air_Resi1_K : Inport  Port=2
  Add : Sum  Inputs=+-
  Constant : Constant  Value=TM_PNT_TMBlock2TMAir_Heat_Resi_KpW
  Divide : Product  Inputs=*/
  Gain : Gain  Gain=-1
  Gain1 : Gain
  PHI_TMBlock_Resi3_W : Outport
  PHI_TM_Air_Resi1_W : Outport  Port=2
  wires:
  Constant/1 -> Divide/2
  Add/1 -> Divide/1
  Divide/1 -> Gain/1, Gain1/1
  Gain/1 -> PHI_TMBlock_Resi3_W/1
  T_TMBlock_Resi3_K/1 -> Add/1
  T_TM_Air_Resi1_K/1 -> Add/2
  Gain1/1 -> PHI_TM_Air_Resi1_W/1

== system METI_CVT_Thermal_ver01_2015a/Vehicle/PTTH_PNT/TMTH_PNT/TMBlock_Heat_Capacity ==
  PHI_TMBlock3_W : Inport
  PHI_TMBlock2_W : Inport  Port=2
  PHI_TMBlock1_W : Inport  Port=3
  PHI_TMBlock4_W : Inport  Port=4
  Add : Sum  Inputs=++++
  Add1 : Sum
  Constant : Constant  Value=TM_PNT_TMBlock_Heat_Capa_JpK
  Constant1 : Constant  Value=TM_PNT_TMBlock_Temp_ini_degC
  Divide : Product  Inputs=/*
  Integrator : Integrator
  degC->K : Subsystem
  T_TMBlock2_K : Outport
  T_TMBlock3_K : Outport  Port=2
  T_TMBlock4_K : Outport  Port=3
  T_TMBlock1_K : Outport  Port=4
  wires:
  PHI_TMBlock2_W/1 -> Add/4
  PHI_TMBlock1_W/1 -> Add/1
  Constant/1 -> Divide/1
  Add/1 -> Divide/2
  Divide/1 -> Integrator/1
  Integrator/1 -> Add1/2
  PHI_TMBlock3_W/1 -> Add/3
  PHI_TMBlock4_W/1 -> Add/2
  Add1/1 -> T_TMBlock1_K/1, T_TMBlock4_K/1, T_TMBlock3_K/1, T_TMBlock2_K/1
  Constant1/1 -> degC->K/1(degC)
  degC->K/1(K) -> Add1/1

== system METI_CVT_Thermal_ver01_2015a/Vehicle/TM_PNT/TC_PNT/LU_Clutch ==
  note: クラッチモデル
      | LockUp ON時は硬いバネダンパー、OFF時はトルク0 Nm
  LockUP_Signal : Inport
  w_TM_PNT_in_radps1 : Inport  Port=2
  w_TM_PNT_in_radps2 : Inport  Port=3
  Gain1 : Gain  Gain=TM_PNT_Gain_LU_spring_Nmprad
  Gain2 : Gain  Gain=TM_PNT_Gain_LU_damper_Nmsprad
  Integrator : Integrator  ExternalReset=level  LimitOutput=on  UpperSaturationLimit=1  LowerSaturationLimit=-1
  Logical Operator : Logic  Operator=NOT  AllPortsSameDT=off  OutDataTypeStr=boolean
  Product : Product  RndMeth=Zero
  Product2 : Product  RndMeth=Zero
  Sum1 : Sum  Inputs=|+-
  Sum2 : Sum  Inputs=++|
  Transfer Fcn : TransferFcn  Denominator=[TM_PNT_tau_LU_Clutch_s 1]
  trq_LUC_Nm1 : Outport
  trq_LUC_Nm2 : Outport  Port=2
  wires:
  w_TM_PNT_in_radps1/1 -> Product/2
  LockUP_Signal/1 -> Logical Operator/1, Transfer Fcn/1
  Sum2/1 -> trq_LUC_Nm2/1, trq_LUC_Nm1/1
  Product2/1 -> Sum1/2
  Product/1 -> Sum1/1
  Integrator/1 -> Gain1/1
  Sum1/1 -> Integrator/1, Gain2/1
  Transfer Fcn/1 -> Product2/1, Product/1
  w_TM_PNT_in_radps2/1 -> Product2/2
  Logical Operator/1 -> Integrator/2
  Gain1/1 -> Sum2/2
  Gain2/1 -> Sum2/1

== system METI_CVT_Thermal_ver01_2015a/Vehicle/TM_PNT/TC_PNT/T_C ==
  w_TM_PNT_in_radps1 : Inport
  w_TM_PNT_in_radps2 : Inport  Port=2
  Cal_C_Capacity : Subsystem
  Cal_Ratio_n : Subsystem
  Cal_trq_TC_eng : Subsystem
  Gain : Gain  Gain=radpsec2rpm
  Gain1 : Gain  Gain=radpsec2rpm
  Product1 : Product  RndMeth=Zero
  トルク比 Lookup Table2 : Lookup_n-D  NumberOfTableDimensions=1  BreakpointsForDimension1=TM_PNT_torque_ratio_table_x_speed_ratio  Table=TM_PNT_torque_ratio_table  ExtrapMethod=Clip  RndMeth=Simplest  InputSameDT=on
  trq_TC_Nm1 : Outport
  trq_TC_Nm2 : Outport  Port=2
  wires:
  Gain/1 -> Cal_Ratio_n/2(n_GR_rpm)  "n_GR_rpm"
  Gain1/1 -> Cal_Ratio_n/1(n_TM_PNT_rpm), Cal_trq_TC_eng/1("n_TM_PNT_rpm ")  "n_TM_PNT_rpm"
  w_TM_PNT_in_radps2/1 -> Gain/1
  Product1/1 -> trq_TC_Nm1/1
  トルク比 Lookup Table2/1 -> Product1/2
  w_TM_PNT_in_radps1/1 -> Gain1/1
  Cal_Ratio_n/1(ratio_n) -> トルク比 Lookup Table2/1, Cal_C_Capacity/1(ratio_n)
  Cal_trq_TC_eng/1(trq_TC_Nm) -> trq_TC_Nm2/1, Product1/1  "trq_TC_Nm"
  Cal_C_Capacity/1(c_capacity) -> Cal_trq_TC_eng/2(c_capacity)
  Cal_Ratio_n/2(flag_acc_del) -> Cal_C_Capacity/2(flag_acc_del)

== system METI_CVT_Thermal_ver01_2015a/Driver/Caliculate_Opeining_Accel/FF/Cal_M_ENG_jiku2/Subsystem ==
  In1 : Inport
  Constant1 : Constant  Value=0
  Switch : Switch  Criteria=u2 > Threshold  Threshold=0.1
  Out1 : Outport
  wires:
  Switch/1 -> Out1/1
  Constant1/1 -> Switch/3
  In1/1 -> Switch/2, Switch/1

== system METI_CVT_Thermal_ver01_2015a/Vehicle/ALT_PNT/Subsystem/I_alt_cal/Cal_I_alt_P_control ==
  note: 目標電圧よりもオルタネータ電圧が低い場合電流をPI制御で出力
      | 高い場合は、電流を0とする
  V_delt_tgt : Inport
  Gain : Gain  Gain=ALT_PNT_Gain_Alt_v_del
  Transfer Fcn : TransferFcn  Denominator=[ALT_PNT_Tau_Alternator_V_tgt_s 1]
  I_alt_base : Outport
  wires:
  Gain/1 -> I_alt_base/1
  V_delt_tgt/1 -> Transfer Fcn/1
  Transfer Fcn/1 -> Gain/1

== system METI_CVT_Thermal_ver01_2015a/Vehicle/ALT_PNT/Subsystem/I_alt_cal/Cal_I_alt_base ==
  note: 目標電圧よりもオルタネータ電圧が低い場合電流をPI制御で出力
      | 高い場合は、電流を0とする
  V_delt_tgt : Inport
  Constant : Constant  Value=0
  Gain : Gain  Gain=1/BT_PNT_Lo_R_lo_batt_ohm
  MinMax : MinMax  Function=max  Inputs=2
  Switch : Switch  Criteria=u2 > Threshold
  Transfer Fcn : TransferFcn  Denominator=[ALT_PNT_Tau_Alternator_V_tgt_s 1]
  I_alt_base : Outport
  wires:
  MinMax/1 -> I_alt_base/1
  Gain/1 -> Switch/1
  V_delt_tgt/1 -> Transfer Fcn/1
  Constant/1 -> MinMax/2, Switch/3
  Switch/1 -> MinMax/1
  Transfer Fcn/1 -> Switch/2, Gain/1

== system METI_CVT_Thermal_ver01_2015a/Vehicle/PTTH_PNT/DFTH_PNT/DFBlock_Heat_Capacity/degC->K ==
  degC : Inport
  Constant2 : Constant  Value=degC2K
  Sum : Sum  Inputs=++|
  K : Outport
  wires:
  degC/1 -> Sum/2
  Constant2/1 -> Sum/1
  Sum/1 -> K/1

== system METI_CVT_Thermal_ver01_2015a/Vehicle/PTTH_PNT/DFTH_PNT/DFOil_Heat_Capacity/degC->K ==
  degC : Inport
  Constant2 : Constant  Value=degC2K
  Sum : Sum  Inputs=++|
  K : Outport
  wires:
  degC/1 -> Sum/2
  Constant2/1 -> Sum/1
  Sum/1 -> K/1

== system METI_CVT_Thermal_ver01_2015a/Vehicle/PTTH_PNT/ENGTH_PNT/Coolant_Heat_Capacity/degC->K ==
  degC : Inport
  Constant2 : Constant  Value=degC2K
  Sum : Sum  Inputs=++|
  K : Outport
  wires:
  degC/1 -> Sum/2
  Constant2/1 -> Sum/1
  Sum/1 -> K/1

== system METI_CVT_Thermal_ver01_2015a/Vehicle/PTTH_PNT/ENGTH_PNT/ENGBlock_Heat_Capacity/degC->K ==
  degC : Inport
  Constant2 : Constant  Value=degC2K
  Sum : Sum  Inputs=++|
  K : Outport
  wires:
  degC/1 -> Sum/2
  Constant2/1 -> Sum/1
  Sum/1 -> K/1

== system METI_CVT_Thermal_ver01_2015a/Vehicle/PTTH_PNT/ENGTH_PNT/ENGOil_Heat_Capacity/degC->K ==
  degC : Inport
  Constant2 : Constant  Value=degC2K
  Sum : Sum  Inputs=++|
  K : Outport
  wires:
  degC/1 -> Sum/2
  Constant2/1 -> Sum/1
  Sum/1 -> K/1

== system METI_CVT_Thermal_ver01_2015a/Vehicle/PTTH_PNT/ENGTH_PNT/ENGOil_Heat_Capacity1/degC->K ==
  degC : Inport
  Constant2 : Constant  Value=degC2K
  Sum : Sum  Inputs=++|
  K : Outport
  wires:
  degC/1 -> Sum/2
  Constant2/1 -> Sum/1
  Sum/1 -> K/1

== system METI_CVT_Thermal_ver01_2015a/Vehicle/PTTH_PNT/RDTH_PNT/ENGBlock2Coolant_Heat_Resistance/K->degC ==
  K : Inport
  Constant2 : Constant  Value=K2degC
  Sum : Sum  Inputs=++|
  degC : Outport
  wires:
  K/1 -> Sum/2
  Constant2/1 -> Sum/1
  Sum/1 -> degC/1

== system METI_CVT_Thermal_ver01_2015a/Vehicle/PTTH_PNT/RDTH_PNT/RDCoolant_Heat_Capacity/degC->K ==
  degC : Inport
  Constant2 : Constant  Value=degC2K
  Sum : Sum  Inputs=++|
  K : Outport
  wires:
  degC/1 -> Sum/2
  Constant2/1 -> Sum/1
  Sum/1 -> K/1

== system METI_CVT_Thermal_ver01_2015a/Vehicle/PTTH_PNT/TMTH_PNT/CVTF_Heat_Capacity/degC->K ==
  degC : Inport
  Constant2 : Constant  Value=degC2K
  Sum : Sum  Inputs=++|
  K : Outport
  wires:
  degC/1 -> Sum/2
  Constant2/1 -> Sum/1
  Sum/1 -> K/1

== system METI_CVT_Thermal_ver01_2015a/Vehicle/PTTH_PNT/TMTH_PNT/TMBlock_Heat_Capacity/degC->K ==
  degC : Inport
  Constant2 : Constant  Value=degC2K
  Sum : Sum  Inputs=++|
  K : Outport
  wires:
  degC/1 -> Sum/2
  Constant2/1 -> Sum/1
  Sum/1 -> K/1

== system METI_CVT_Thermal_ver01_2015a/Vehicle/TM_PNT/TC_PNT/T_C/Cal_C_Capacity ==
  note: 容量係数
      | 加速中は＋
      | 減速中は－
  note: capacity coefficient
  note: N・m/rpm2
  ratio_n : Inport
  flag_acc_del : Inport  Port=2
  Product2 : Product  RndMeth=Zero
  ×10＾-6 : Gain  Gain=TM_PNT_ConvUnit
  容量係数 Lookup Table1 : Lookup_n-D  NumberOfTableDimensions=1  BreakpointsForDimension1=TM_PNT_torque_capacity_Nmprpm2_table_x_speed_ratio  Table=TM_PNT_torque_capacity_Nmprpm2_table  RndMeth=Simplest  InputSameDT=on
  c_capacity : Outport
  wires:
  容量係数 Lookup Table1/1 -> ×10＾-6/1
  ×10＾-6/1 -> Product2/1
  ratio_n/1 -> 容量係数 Lookup Table1/1
  Product2/1 -> c_capacity/1
  flag_acc_del/1 -> Product2/2

== system METI_CVT_Thermal_ver01_2015a/Vehicle/TM_PNT/TC_PNT/T_C/Cal_Ratio_n ==
  n_TM_PNT_rpm : Inport
  n_GR_rpm : Inport  Port=2
  Compare To Constant1 : simulink/Logic and Bit Operations/Compare To Constant  relop=<=  const=TM_PNT_n_TC_min_rpm  OutDataTypeStr=boolean
  Compare To Constant2 : simulink/Logic and Bit Operations/Compare To Constant  relop=<=  const=TM_PNT_n_TC_min_rpm  OutDataTypeStr=boolean
  Constant : Constant  Value=0
  Logical Operator1 : Logic  Operator=OR  AllPortsSameDT=off  OutDataTypeStr=boolean
  MinMax : MinMax  Inputs=2
  Saturation1 : Saturate  UpperLimit=TM_PNT_w_ROT_T_C_UL  LowerLimit=TM_PNT_w_ROT_T_C_LL
  Saturation2 : Saturate  UpperLimit=TM_PNT_w_ROT_T_C_UL  LowerLimit=TM_PNT_w_ROT_T_C_LL
  Saturation5 : Saturate  UpperLimit=TM_PNT_ratio_w_ROT_T_C_UL  LowerLimit=TM_PNT_ratio_w_ROT_T_C_LL
  Subsystem : Subsystem
  Switch : Switch  Threshold=0.5
  加速時速度比 : Product  Inputs=*/
  減速時速度比 : Product  Inputs=*/
  ratio_n : Outport
  flag_acc_del : Outport  Port=2
  wires:
  Saturation2/1 -> 減速時速度比/1, 加速時速度比/2
  Saturation1/1 -> 減速時速度比/2, 加速時速度比/1
  加速時速度比/1 -> MinMax/1
  減速時速度比/1 -> MinMax/2
  MinMax/1 -> Saturation5/1
  Saturation5/1 -> Switch/3
  Constant/1 -> Switch/1
  Compare To Constant2/1 -> Logical Operator1/1
  Compare To Constant1/1 -> Logical Operator1/2
  Logical Operator1/1 -> Switch/2
  Switch/1 -> ratio_n/1
  n_GR_rpm/1 -> Subsystem/2(omg_tm), Saturation1/1, Compare To Constant1/1  "omg_tm"
  n_TM_PNT_rpm/1 -> Compare To Constant2/1, Subsystem/1(omg_engine), Saturation2/1  "omg_engine"
  Subsystem/1(flag_acc_del) -> flag_acc_del/1

== system METI_CVT_Thermal_ver01_2015a/Vehicle/TM_PNT/TC_PNT/T_C/Cal_trq_TC_eng ==
  "n_TM_PNT_rpm " : Inport
  c_capacity : Inport  Port=2
  Math Function : Math  Operator=magnitude^2  SaturateOnIntegerOverflow=on
  Product : Product  RndMeth=Zero
  trq_TC_Nm : Outport
  wires:
  Product/1 -> trq_TC_Nm/1
  Math Function/1 -> Product/1
  c_capacity/1 -> Product/2
  "n_TM_PNT_rpm "/1 -> Math Function/1

== system METI_CVT_Thermal_ver01_2015a/Vehicle/TM_PNT/TC_PNT/T_C/Cal_Ratio_n/Subsystem ==
  note: エンジン加速中は1、減速中は-1
  omg_engine : Inport
  omg_tm : Inport  Port=2
  Saturation : Saturate  UpperLimit=1  LowerLimit=-1
  Subtract : Sum  Inputs=-+|
  flag_acc_del : Outport
  wires:
  Subtract/1 -> Saturation/1
  Saturation/1 -> flag_acc_del/1
  omg_tm/1 -> Subtract/1
  omg_engine/1 -> Subtract/2
